simulink model "AirRefueling_Platform_IBVS"  (R2022b)
settings: Solver=FixedStepAuto  StartTime=0.0  StopTime=70  FixedStep=0.02  RelTol=1e-5  AbsTol=1e-4  EnableMultiTasking=on
InitFcn:
  | F16_Init
values from neighbouring files (symbols this model uses):
  airSpeed = 393.720000000000    (= 393.72)    [F16_Init.m]    (also in Initialization.m)
  alpha0 = trimAlpha*180/pi    (= 6.62393794015)    [F16_Init.m]    (also in Initialization.m)
  altitude = 9843    [F16_Init.m]    (also in Initialization.m)
  b_ref = 30.0    (= 30)    [F16_Init.m]    (also in Initialization.m)
  C2m = [C(1,:) ... (first row only)    [F16_Init.m]    (also in Initialization.m)
  d_f_rc = [3.75;0;-0.86]    [F16_Init.m]
  d_pr_rc = [6.06;0.54;-0.86]    [F16_Init.m]
  dLEF = 0    [F16_Init.m]    (also in Initialization.m)
  fi_flag = 1    [F16_Init.m]    (also in Initialization.m)
  Kc = [ ... (first row only)    [F16_Init.m]    (also in Initialization.m)
  Ki = zeros(4,3)    [F16_Init.m]    (also in Initialization.m)
  Kp = zeros(4,18)    [F16_Init.m]    (also in Initialization.m)
  mass = 636.94    [F16_Init.m]    (also in Initialization.m)
  p0_rc = [-14.35-6.06-6;-0.54-(2);5.12+0.86-(-2)]    [F16_Init.m]
  q = zeros(N,1)    [hose3D_n_air_Fv_correction.m]
  trim_ail = 0.00874607850103852    (= 0.00874607850104)    [F16_Init.m]    (also in Initialization.m)
  trim_control = [trim_thrust;trim_ele;trim_ail;trim_rud]    [F16_Init.m]    (also in Initialization.m)
  trim_ele = -2.97973164860638    (= -2.97973164861)    [F16_Init.m]    (also in Initialization.m)
  trim_rud = 0.0680302158182712    (= 0.0680302158183)    [F16_Init.m]    (also in Initialization.m)
  trim_state1 = [trim_state;0;0;0;0;0;0]    [F16_Init.m]    (also in Initialization.m)
  trim_thrust = 2279.08519954656    (= 2279.08519955)    [F16_Init.m]    (also in Initialization.m)
undefined symbols (not defined in the file or in its folder): F, gray, MIL, vt0
libraries: aerolibconvert2 x4, aerolibasang x4, aerolibwind2 x3, visionmorphops x3, vrlib x2, aerolibobsolete x2, simulink x1, visionconversions x1, visiongeotforms x1, aerolibatmos2 x1, aerolibadyn x1, aerolibanimutils x1
(part 2 of 2)

== matlab function AirRefueling_Platform_IBVS/Visual Servo Block/MATLAB Function1 ==
  settings: updateMethod=DISCRETE
  data: u1 input; yy output; u2 input; u3 input; yy1 output; yy2 output; t input; AA data_store_memory; yytest output
%function [yy,yy1,yy2,posNdepth] = fcn(u1,u2,u3,t)
function [yy,yy1,yy2,yytest] = fcn(u1,u2,u3,t)
%#codegen
L=u1; %过滤后图像
N=u2; %识别出的目标点个数
Ir=u3; %原灰度图像
t0=0.1;
global AA;
%S=zeros(N,2);
dX=zeros(10,1);
dY=zeros(10,1);
 for k=1:N    %对所有出现的标志点进行计算，获得每个标志点图像坐标系下横纵坐标的平均下标位置。
     [r,c]=find(L == k);
     dX(k)=mean(r);   %r行数，也就是y坐标
     dY(k)=mean(c);   %c列数，也就是x坐标
 end
% %plot(S(:,1),S(:,2),'+')
% % dx(:,1)=S(:,1)-mean(S(:,1));
% % dy(:,1)=S(:,2)-mean(S(:,2));
% 
% dX=S(:,1);
% dY=S(:,2);

m=[dX(1:N,1) dY(1:N,1) ones(size(dX(1:N,1)))]\-(dX(1:N,1).^2+dY(1:N,1).^2);
% m = [dX(1:N,1) dY(1:N,1) ones(size(dX(1:N,1)))]的逆* -(dX(1:N,1).^2+dY(1:N,1).^2)
cX=-0.5*m(1);%目标锥套的圆心图像坐标以及半径（以左上点为坐标系原点的像素坐标系下的坐标以及半径长度）
cY=-0.5*m(2);
cR=sqrt((m(1)^2+m(2)^2)/4-m(3));%半径
if N==3
   AA=[cX;cY;cR]; 
end

if N<3
   cX=AA(1);
   cY=AA(2);
   cR=AA(3);
end

%yy=N;
% 
%yy = [cX,cY,cR];
%yy=[yy,N];


[mm,nn]=size(Ir);%图像视野大小  mm代表像素行数，nn代表像素列数。
%因为这里图像坐标系下横轴是x，纵轴是y。因此这里nn就是图像坐标系x轴坐标，mm就是图像坐标系y轴坐标。


if t>t0
    alpha=0:pi/100:2*pi;
    x=cR*cos(alpha)+cX;
    y=cR*sin(alpha)+cY;

    % if isempty(Ir)
    %     Ir=zeros(720,1280);    
    % end





    for k=1:length(alpha)

        i=floor(x(k));%取整
        j=floor(y(k));
        if(i>=1&&j>=1&&i<=mm&&j<=nn)
            Ir(i:i,j:j)=1;        
        end

    end
end    
    
if t>t0+0.05
    i=floor(cX);
    j=floor(cY);

    if(i-3>=1&&j-3>=1&&i+4<=mm&&j+4<=nn)
        Ir(i-3:i+4,j:j+1)=1; 
        Ir(i:i+1,j-3:j+4)=1;  
    end
end

if t>t0+0.1
    i=floor(mm/2+42.57);
    j=floor(44.14+nn/2);
    if(i-3>=1&&j-3>=1&&i+4<=mm&&j+4<=nn)
        Ir(i-3:i+4,j:j+1)=1; 
        Ir(i:i+1,j-3:j+4)=1;  
    end
end

yy=Ir;
% 
% 
% 
% 

yy1=[cY-nn/2,mm/2-cX,cR]; 
%yy1 以图像中心为原点的图像坐标系下的X,Y位置以及图像中半径长度。 这些均为像素长度，也就是矩阵里的下标个数。
%因为这里图像坐标系的y轴是向下的，因此这里yy1的y坐标就是mm/2-cX而不是cX-mm/2


%从像素坐标系转化为相机坐标系，相机坐标系下，x轴指向机头，y轴是图像坐标系下的x轴，z轴是图像坐标系下的y轴，因此这里有
%xw<-cR(yy1(2)), yw<-x(yy1(0)), zw<-y(yy1(1)).

f=196.8372/0.330;
s=196.8372/yy1(3);
xw=-s+1.928; %锥套的深度信息
yw=yy1(1)*s/f-(46.94*1.862225/f);
zw=yy1(2)*s/f+(52.06*1.862225/f)-0.02;



%ftest=196.8372/0.330;
xtest=s-1.928; %实际仿真最后对接成功，深度就是大约2.3.   这里的1.928是什么？
ytest=yy1(1)*s/f-(46.94*1.862225/f);
ztest=-(yy1(2)*s/f+(52.06*1.862225/f));
yytest=[xtest,ytest,ztest];

yyw=-yw;
xxw=xw*cos(5/180*pi)-zw*sin(5/180*pi);
zzw=xw*sin(5/180*pi)-zw*cos(5/180*pi);

% xw=-s+1.8925;
% 
% yw=(yy1(1)*s/2/196.9344-0.2206)/-1.4705;
% zw=(yy1(2)*s/2/196.9344+0.4953-2.9364-1.4682*xw)/1.4682;
yy2=[xxw;yyw;zzw];
posNdepth=[xw;yw;zw];
% yy2=[xw;yw;zw];


% function [yy,yy1,yy2] = fcn(u1,u2,u3)
% %#codegen
% L=u1;
% N=u2;
% Ir=u3;
% %S=zeros(N,2);
% dX=zeros(10,1);
% dY=zeros(10,1);
%  for k=1:N
%      [r,c]=find(L == k);
%      dX(k)=mean(r);
%      dY(k)=mean(c);     
%  end
% % %plot(S(:,1),S(:,2),'+')
% % % dx(:,1)=S(:,1)-mean(S(:,1));
% % % dy(:,1)=S(:,2)-mean(S(:,2));
% % 
% % dX=S(:,1);
% % dY=S(:,2);
% 
% m=[dX(1:N,1) dY(1:N,1) ones(size(dX(1:N,1)))]\-(dX(1:N,1).^2+dY(1:N,1).^2);
% cX=-0.5*m(1);
% cY=-0.5*m(2);
% cR=sqrt((m(1)^2+m(2)^2)/4-m(3));
% 
% 
% %yy=N;
% % 
% %yy = [cX,cY,cR];
% %yy=[yy,N];
% 
% % 
% alpha=0:pi/100:2*pi;
% x=cR*cos(alpha)+cX;
% y=cR*sin(alpha)+cY;
% 
% % if isempty(Ir)
% %     Ir=zeros(720,1280);    
% % end
% 
% [mm,nn]=size(Ir);
% for k=1:length(alpha)
% 
%     i=floor(x(k));
%     j=floor(y(k));
%     if(i>=1&&j>=1&&i<=mm&&j<=nn)
%         Ir(i:i,j:j)=1;        
%     end
%         
% end
% 
% i=floor(cX);
% j=floor(cY);
% 
% if(i-3>=1&&j-3>=1&&i+4<=mm&&j+4<=nn)
%     Ir(i-3:i+4,j:j+1)=1; 
%     Ir(i:i+1,j-3:j+4)=1;  
% end
% 
% % 
% % 
% % 
% % 
% yy=Ir;
% 
% yy1=[cY-nn/2,mm/2-cX,cR];
% 
% s=196.9344/yy1(3);
% xw=-s+1.8925;
% 
% yw=(yy1(1)*s/2/196.9344-0.2206)/-1.4705;
% zw=(yy1(2)*s/2/196.9344+0.4953-2.9364-1.4682*xw)/1.4682;
% yy2=[xw;yw;zw];
% 
%

== matlab function AirRefueling_Platform_IBVS/Visual Servo Block/MATLAB Function2 ==
  data: u input; y output
function y = fcn(u)
%#codegen

Ir=u(:,:,2)*2-u(:,:,1)*1-u(:,:,3)*1;

S=size(Ir);
Iin=zeros(S(1),S(2));
for i=1:S(1)
    for j=1:S(2)
       if Ir(i,j)<50
            Iin(i,j)=0;
        else
            Iin(i,j)=1;
       end
        
       if i/S(1)>0.8
           Iin(i,j)=0;
       end
       
    end
end


y = Iin;

== matlab function AirRefueling_Platform_IBVS/Visual Servo Block/MATLAB Function3 ==
  data: u1 input; yy output; u2 input; u3 input; t input
function yy = fcn(u1,u2,u3,t)
%#codegen
L=u1;
N=u2;
Ir=u3;
t0=0.25;
%S=zeros(N,2);
dX=zeros(10,1);
dY=zeros(10,1);


 for k=1:N
     [r,c]=find(L == k);
     dX(k)=mean(r);
     dY(k)=mean(c);     
 end
% %plot(S(:,1),S(:,2),'+')
% % dx(:,1)=S(:,1)-mean(S(:,1));
% % dy(:,1)=S(:,2)-mean(S(:,2));
% 
% dX=S(:,1);
% dY=S(:,2);
[mm,nn]=size(Ir);

if N==6
   [dX_up,I]=min(dX(1:6));
   

   
   if t>t0
   aa=dX(I)-mean([dX(1:I);dX(I+1:6)]);
   bb=(max(dY(1:6))-min(dY(1:6)))/6;
   
   if abs(aa/bb)>0.2

       for i=1:6
           if(i~=I)
               for j=1:29
                   i1=floor(dX(I)+(dX(i)-dX(I))/30*j);
                   j1=floor(dY(I)+(dY(i)-dY(I))/30*j);  
                   if(i1>=1&&j1>=1&&i1<=mm&&j1<=nn)              
                       Ir(i1:i1,j1:j1)=1;         
                   end             
               end    
           end       
       end          
   
   end       
       
       

   end
   dX(I:9)=dX(I+1:10); 
   dY(I:9)=dY(I+1:10);    
end

if t>t0+0.05
    ll=4;
    if N==4
       ll=3; 
    end
    if N>6
       ll=4;
    end
    
    for i=1:ll
       for j=1:19
           i1=floor(dX(i)+(dX(i+1)-dX(i))/20*j);
           j1=floor(dY(i)+(dY(i+1)-dY(i))/20*j);  
           if(i1>=1&&j1>=1&&i1<=mm&&j1<=nn)              
               Ir(i1:i1,j1:j1)=1;         
           end             
       end          
    end     
end

% 
% 
% 
% m=[dX(1:N,1) dY(1:N,1) ones(size(dX(1:N,1)))]\-(dX(1:N,1).^2+dY(1:N,1).^2);
% cX=-0.5*m(1);
% cY=-0.5*m(2);
% cR=sqrt((m(1)^2+m(2)^2)/4-m(3));
% 
% 
% %yy=N;
% % 
% %yy = [cX,cY,cR];
% %yy=[yy,N];
% 
% % 
% alpha=0:pi/100:2*pi;
% x=cR*cos(alpha)+cX;
% y=cR*sin(alpha)+cY;
% 
% % if isempty(Ir)
% %     Ir=zeros(720,1280);    
% % end
% 
% [mm,nn]=size(Ir);
% for k=1:length(alpha)
% 
%     i=floor(x(k));
%     j=floor(y(k));
%     if(i>=1&&j>=1&&i+1<=mm&&j+1<=nn)
%         Ir(i:i+1,j:j+1)=1;        
%     end
%         
% end
% 
% i=floor(cX);
% j=floor(cY);
% 
% if(i-3>=1&&j-3>=1&&i+4<=mm&&j+4<=nn)
%     Ir(i-3:i+4,j:j+1)=1; 
%     Ir(i:i+1,j-3:j+4)=1;  
% end
% 
% % 
% 
% 
% 
yy=Ir;

== matlab function AirRefueling_Platform_IBVS/Visual Servo Block/MATLAB Function4 ==
  data: u1 input; y output; u2 input
function y = fcn(u1,u2)
%#codegen

%y = u1;
y = u1+u2;

== matlab function AirRefueling_Platform_IBVS/Receiver System/Controller/IBVS Conroller ==
  data: Z input; ex input; ey input; u_vcz output; u_vcy output; u_vcx output; F16State input
function [u_vcz,u_vcy,u_vcx] = fcn(Z,ex,ey, F16State)

ey = -ey;%坐标系转换需要变号。

%% 对接成功，参数也对。
Z_d = 2.0;

% kz = 0.3;
kz = 0.5;
% ky = 2;
ky = 3;

k1 = 3; k2 = 1;
% u_vcz = kz*(Z-Z_d)-k1*(abs(ex))-k2*(abs(ey))-F16State(10,1)*0.86+F16State(12,1)*0.54;
u_vcz = kz*(Z-Z_d)-k1*(abs(ex)/abs(Z))-k2*(abs(ey)/abs(Z))-F16State(10,1)*0.86+F16State(12,1)*0.54;
u_vcy = ky*(ey-0)-F16State(10,1)*0.54+F16State(11,1)*6.06;

kx = 1;
u_vcx = kx*(ex-0)-F16State(12,1)*6.06+F16State(10,1)*0.86;


%% 利用迭代学习的前向速度控制，使用图像误差缩小横竖误差，这里可以对接成功。
% ky = 3;
% u_vcy = ky*(ey-(0.5));
% kx = 1;
% u_vcx = kx*(ex-0);



%% 第二次控制实验：加入头波的影响后，当前参数也可以完成对接。此时头波大小在仿真里为1倍。
% %10倍头波在此参数下只能接近，不能对接成功。
% Z_d = 2.0;
% kz = 0.5;
% ky = 5;
% 
% 
% k1 = 3; k2 = 1;
% % u_vcz = kz*(Z-Z_d)-k1*(abs(ex))-k2*(abs(ey));
% u_vcz = kz*(Z-Z_d)-k1*(abs(ex)/abs(Z))-k2*(abs(ey)/abs(Z));
% u_vcy = ky*(ey-0);
% 
% kx = 1.6;
% u_vcx = kx*(ex-0);


% Z_d = 2.0;
% kz = 0.5;
% ky = 2;
% 
% k1 = 3; k2 = 1;
% % u_vcz = kz*(Z-Z_d)-k1*(abs(ex))-k2*(abs(ey))-F16State(10,1)*0.86+F16State(12,1)*0.54;
% u_vcz = kz*(Z-Z_d)-k1*(abs(ex)/abs(Z))-k2*(abs(ey)/abs(Z))-F16State(10,1)*0.86+F16State(12,1)*0.54;
% u_vcy = ky*(ey-0)-F16State(10,1)*0.54+F16State(11,1)*6.06;
% 
% kx = 1;
% u_vcx = kx*(ex-0)-F16State(12,1)*6.06+F16State(10,1)*0.86;

== matlab function AirRefueling_Platform_IBVS/Receiver System/F16 Nonlinear Model/Environment Models/mass variable ==
  data: g input; y output; mass input; time input
function y = fcn(g,mass,time)

if(time<50)
    y = mass*g;
else
    y = (mass+(time-50)*2)*g
end

== matlab function AirRefueling_Platform_IBVS/Hose-Drogue System/HDU Function ==
  data: t input; u input; y3 output; dp input
function y3  = fcn(t,u,dp)
% persistent hwpState;
% if isempty(hwpState)
%     hwpState=zeros(20,1);
% end

ll=zeros(20,1);
for i=1:20
    if i==1
       uk_1 = [0;0;0];
    else
        uk_1 = [u(3*(i-1)-2);u(3*(i-1)-2+1);u(3*(i-1)-2+2)];
    end
    uk = [u(3*(i)-2);u(3*(i)-2+1);u(3*(i)-2+2)];
    
    ll(i)=sqrt((uk(1)-uk_1(1))^2+(uk(2)-uk_1(2))^2+(uk(3)-uk_1(3))^2);
end

y = sum(ll);

y1= sqrt((u(58))^2+(u(59))^2+(u(60))^2);
y2 = y1-y;

y3  = 0;

% hwpState = [((y1/14.29*14.33-y)/y);hwpState(1:19)];

% rolldown = true;
% for i=1:20
%     if hwpState(i)<-0.0005
%         rolldown =false;
%         break;
%     end
% end

rolldown = false;
if dp(1)<-0.3 && ((y1/14.29*14.33-y)/y) >=-0.001
    rolldown = true;
end

if rolldown
    y3=sat((y-14.33)/1)*1*1.2;
else
    y3=0;
    if ((y1/14.29*14.33-y)/y) <=-0.01
        y3 = -4*(y1/14.29*14.33-y);
    elseif ((y1/14.29*14.33-y)/y) <=-0.0015
        y3 = -2*(y1/14.29*14.33-y);
%     elseif((y1/14.29*14.33-y)/y) <=-0.0015
%         y3 = -3*(y1/14.29*14.33-y);
    end    
end




% elseif ((y1/14.29*14.33-y)/y) >=-0.001
%     y3=sat((y-14.33)/0.8)*0.8*0.8;
% end


if t<12
    y3=0;
end

y2=(y1/14.29*14.33-y)/y;

== matlab function AirRefueling_Platform_IBVS/Hose-Drogue System/Subsystem/MATLAB Function ==
  data: u input; y output
function y = fcn(u)
y=0;

if u<=3
    y=14;
end
if u<=13 && u>3
    y=14-((u-3)*14/10);
end

== matlab function AirRefueling_Platform_IBVS/Hose-Drogue System/Collision Model ==
  settings: updateMethod=DISCRETE
  data: u input; y output; v input
function y = fcn(u,v)

u(1) = u(1)-0.1; % Redefine the drogue center.

persistent isXCrossBound;
if isempty(isXCrossBound)
    isXCrossBound = false;
end

persistent isRCrossBound;
if isempty(isRCrossBound)
    isRCrossBound = false;
end


persistent lastPosState;
if isempty(lastPosState)
    lastPosState = [0;0;0];
end


if ~isXCrossBound && lastPosState(1)<=0 && u(1)>0
    isXCrossBound =true;
end

if isXCrossBound&& u(1)<-0.05 && lastPosState(1) >= -0.05
    isXCrossBound=false;
end


R = sqrt(u(2)^2+u(3)^2);
RLast = sqrt(lastPosState(2)^2+lastPosState(3)^2);

RDrogue = 0.2;
 if u(1)>-0.15 && u(1)<0
     RDrogue = 0.1*(-u(1)/0.15)+0.1;
 end
 
 if u(1)>=0
     RDrogue = 0.1;
 end


if ~isRCrossBound &&  R>(RDrogue+0.015) && u(1)>-0.1 && (u(1)<=0 || isXCrossBound) && RLast <=(RDrogue+0.01)
    isRCrossBound = true;
end

if isRCrossBound  && R<RDrogue && u(1)>-0.15 && (u(1)<=0 || isXCrossBound) && RLast>=RDrogue
    isRCrossBound = false;
end

if isRCrossBound && u(1)<=-0.15 && ~isXCrossBound
    isRCrossBound = false;
end


y=[0;0;0];


if isXCrossBound
    if u(1) <0.05
        y(1)=2000*u(1);
        if v(1)>0
            y(1) = y(1) + 1000*v(1);
            y(2)=600*v(2);
            y(3)=600*v(3);
        end  
    else
         y(1) = 1000*u(1)+3000*v(1);
         y(2)=200*v(2);
         y(3)=200*v(3);         
    end 
end

eR = R - RDrogue;
if ~isXCrossBound && u(1)>-0.1 && u(1)<=0.1 && eR<=0 
      y(2)=200*v(2);
      y(3)=200*v(3); 
end


if isRCrossBound
    if eR < 0.05
        Ru = 5000*eR;
        y(2) = Ru*u(2)/R;
        y(3) = Ru*u(3)/R;
        if R>RLast
            y(2) = y(2)+ 200*v(2);
            y(3) = y(3)+ 200*v(3);
        end
    else
            Ru = 10000*eR;
            y(2) = Ru*u(2)/R+50*v(2);
            y(3) = Ru*u(3)/R+50*v(3);              
    end
end

lastPosState = u;


%y=[0;0;0];
% if u(1)<-0.1 && (u(2) > 0.05)

% if u(1)>0 && v(1)>0
% %     if v(1)>=1
% %         y(1)=1000*v(1);
% %         if(u(1)>0.05)
% %             y(1)= y(1)+10000*u(1);
% %         end
% %     else
% %         if(u(1)>0.05)
% %             y(1)=10000*u(1);
% %         else
% %             y(1)=500*u(1)+100*v(1);
% %         end 
% %     end
%     y(1)=1000*u(1);
%     if u(1)>0.01
%         y(1)=2000*u(1);
%     end
%     
%     if u(1)>0.02
%         y(1)=5000*u(1);
%     end  
%     %y(1)=y(1)+100*v(1);
%     
% end


% if u(1)>-0.1 && u(2) > 0.05 %&& u(2) <0.08
%     y(2)=5000*(u(2)-0.05);
% end
% 
% if u(1)>-0.1 && u(2) <- 0.05 %&&  u(2) >- 0.08
%     y(2)=5000*(u(2)+0.05);
% end
% 
% if u(1)>-0.1 && u(3) > 0.05 %&&  u(3) < 0.08
%     y(3)=5000*(u(3)-0.05);
% end
% 
% if u(1)>-0.1 && u(3) <- 0.05 %&& u(3) >- 0.08
%     y(3)=5000*(u(3)+0.05);
% end




% if u(1)>-0.15 && u(3) > 0.2
%     if v(3)>=1
%         y(3)=1000*v(3);
%     else
%         y(3)=5000*(u(3)-0.2)+100*v(3);
%     end
% end
% 
% if u(1)>-0.15 && u(3) <- 0.2
%     if v(3)<=-1
%         y(3)=1000*v(3);
%     else
%         y(3)=5000*(u(3)+0.2)+100*v(3);
%     end
% end

== matlab function AirRefueling_Platform_IBVS/Tanker System/  ==
  data: u input; y output

function y = WindTurFromTank(u)
%#codegen

%横纵向气流角速度等下计算长度
c_lat=4;
c_lon=4;

%两端参考点
u1 = u+[0 ,c_lat ,0]';
u2 = u+[0 ,-c_lat, 0]';

yy1 = TankerVortexWindField(u1);
yy2 = TankerVortexWindField(u2);

%计算x轴向滚转角速度
yp = (yy1(3) - yy2(3))/4/c_lat;

u3=u+[c_lon, 0,0]';
u4=u+[-c_lon ,0,0]';
yy3 = TankerVortexWindField(u3);
yy4 = TankerVortexWindField(u4);

%俯仰角速度计算
yq = -(yy3(3) - yy4(3))/4/c_lon;

%偏航角速度设为0
yr = 0;

%质心处风场计算
y_uvw = TankerVortexWindField(u);


%y = [y_uvw(1);y_uvw(2);y_uvw(3);-yp;-yq;-yr]*0.5;
y = [y_uvw(1);y_uvw(2);y_uvw(3);-yp;-yq;-yr];

== matlab function AirRefueling_Platform_IBVS/SimToVR1 ==
  data: t input; y output; PosPr1 input; PosTb1 input
function y = SimToVR(t,PosPr1,PosTb1)
%#codegen

%%函数名：SimToVR
%%用途  ：将软管锥套坐标输出转换为VR输入
%%输入  ：PosPr - 受油机椎管坐标， PlsTb - 软管坐标数据
%%输出  ：VrPos - 软管和受油机VR位置，VrAngle - 旋转角度输出
%%作者  ：戴训华
%%时间  ：2014/3/19

PosPr = PosPr1(1:3);
AttitudeRecei = [PosPr1(4);-PosPr1(6);PosPr1(5)-0.115609];

PosTb = PosTb1(1:60);

VrAngle = zeros(22*4,1);
VrPos = zeros(22*3,1);


for j = 1:21                        %前20为软管坐标数据，后1为软管平滑过渡处理
    if j == 1
        pX = [0, 0, 0]';            %软管起点
        pY = PosTb(3*j-2:3*j);      %软杆终点
    elseif j == 21                  %多加一段杆，做过渡
        pX = PosTb(3*j-5:3*j-3);
        pY = [PosTb(3*j-5)-0.7163*cos(8/180*pi),PosTb(3*j-4),PosTb(3*j-3)+0.7163*sin(8/180*pi)]';
    else
        pX = PosTb(3*j-5:3*j-3);
        pY = PosTb(3*j-2:3*j); 
    end
    
    pZ = (pX + pY)/2;               %中点坐标
    pZ = pZ * 8/3;                  %到VR中比例的缩放

    vAxis = [0,0,-1]';               %水平轴
    vTb = pY - pX;                  %杆的方向
    
    axis1 = null([vAxis';vTb']);%获取垂直向量
    vRot = axis1(:,1)';             %得到旋转轴
    
    if vRot(2) < 0
        vRot = -vRot;
    end
    
    VrAngle(4*j-3:4*j-1) = [vRot(1),vRot(3),vRot(2)]';
    VrAngle(4*j) = acos(vAxis'*vTb / sqrt(vAxis'*vAxis * vTb'*vTb));
    
    VrPos(3*j-2:3*j) = [pZ(1),-pZ(3),pZ(2)]';
end
%y = u;
VrAngle(85:88)=[AttitudeRecei(1);AttitudeRecei(2);AttitudeRecei(3);norm(AttitudeRecei)];
pZ = PosPr+[0.35 -0.1 -0.05]';
pZ = pZ * 8/3;
VrPos(3*22-2:3*22) = [pZ(1),-pZ(3),pZ(2)]';

VrPos(3*21-2) = VrPos(3*21-2)+0.8;
VrPos(3*21-1) = VrPos(3*21-1)+0.1;

if t<10
    if t>1
        VrPos(1:21*3) = VrPos(1:21*3)*(t-1)/9;
    else
        VrPos(1:21*3) = VrPos(1:21*3)*0;
    end
end

y = [VrAngle;VrPos];

== matlab function AirRefueling_Platform_IBVS/Original IBVS/MATLAB Function ==
  data: image input; dis output; t input; Num_image input; flag output
function [dis,flag] = fcn(image,t,Num_image)
coder.extrinsic('imwrite');
coder.extrinsic('fullfile');
coder.extrinsic('assignin');

flag=0;
    if t>2.9 && t<6.1
%         Num_image=Num_image+1;
        title=int2str(Num_image);
        title=[title,'.jpg'];
        imagepath="E:\image tracking\Simulation";
        filename=fullfile(imagepath,title);
        imwrite(image,filename); 
        assignin('base','Num_image',Num_image);
        flag=1;
        
%         imsave(image);
%         video = VideoWriter('E:\image tracking\Simulation\Simulation.avi');
%         open(video);
%         writeVideo(video,image)
%         close(video);
    end
    dis=Num_image;
end

== matlab function AirRefueling_Platform_IBVS/Hose-Drogue System/Bow Wave Effect/Bow Wave Effect Function ==
  data: x input; Fx output; y input; z input; Fy output; Fz output
function [Fx,Fy,Fz] = F_rc2dr(x,y,z)

Cx1 = 91.6170;
Cx2 = 0.3220;
Cx3 = 3.8870;
Cx4 = 2.7359;
Cx5 = 2.4939;
Cx6 = 309.7709;
Cx7 = 0.3237;
Cx8 = 0.3851;
Cx9 = 1.1471;

Cy1 = 223.3210;
Cy2 = 0.2082;
Cy3 = 0.8102;
Cy4 = 0.6555;

Cz1 = 173.2021;
Cz2 = 0.2141;
Cz3 = 0.5697;
Cz4 = 0.7038;

if x > 5.6493
    Fx = 0;
elseif x > 3.0893
    Fx = Cx1*(1-Cx2*(x-Cx3)^2)*exp(-y^2/Cx4)*exp(z/Cx5);
else
    Fx = Cx1*(1-Cx2*(x-Cx3)^2)*exp(-y^2/Cx4)*exp(z/Cx5)...
       + Cx6*(1-Cx7*x)*exp(-y^2/Cx8)*exp(z/Cx9);
end

if x > 4.8031
    Fy = 0;
else
    Fy = Cy1*(1-Cy2*x)*(y*exp(-y^2/Cy3))*exp(z/Cy4);
end

if x > 4.6275
    Fz = 0;
else
    Fz = -Cz1*(1-Cz2*x)*exp(-y^2/Cz3)*exp(z/Cz4);
end

== matlab function AirRefueling_Platform_IBVS/Hose-Drogue System/Total Turbulence   ==
  data: u1 input; u input; y output
function y = Dr_wnd2Frc(u1,u)
%#codegen

Ve=120;
rho = 0.98;
Q=0.5*rho*Ve^2;
S=0.38;
CD=0.81*0.8;

uu=u(1);
vv=u(2);
ww=u(3);

%beta = acos(sqrt(vv^2+ww^2)/abs(uu));
%theta = atan(ww/vv);

C_beta = 0.3979;

yx=rho*S*CD*Ve*uu;
yy=Q*S*C_beta*vv/Ve;
yz=Q*S*C_beta*ww/Ve;


y = [yx,yy,yz]';
y=u1+y;

== matlab function AirRefueling_Platform_IBVS/Original IBVS/MATLAB Function1 ==
  data: image input; bw_image output
function bw_image = fcn(image)
row=200;col=320;
for i=1:row
    for j=1:col
        if image(i,j,1)>0.5 && image(i,j,2)<0.1 && image(i,j,3)<0.1
            image(i,j,:)=1;
        else
            image(i,j,:)=0;
        end
    end
end
gray=rgb2gray(image);

bw_image =imbinarize(gray);

== matlab function AirRefueling_Platform_IBVS/Original IBVS/MATLAB Function2 ==
  data: label_image input; ey output; cout input; ex output
function [ey,ex] = fcn(label_image,cout)
row=200;col=320;x=0;n_x=0;y=0;n_y=0;
i=1;j=1;
for i=1:row
    for j=1:col
        if label_image(i,j)==1
        x=x+i;y=y+j;
        n_x=n_x+1;n_y=n_y+1;
        end
    end
end
ey=x/n_x-row/2;
ex=y/n_y-col/2;
end
